simulink model "dqtransform2"  (R2014b)
settings: Solver=ode45  StartTime=0.0  StopTime=10  MaxStep=1e-4  RelTol=1e-3
undefined symbols (not defined in the file): f, Vg
settings Model: Creator=Iranga Weerasuriya  LastModifiedBy=ajunyent
settings DataIOCC: SignalLoggingSaveFormat=ModelDataLogs
settings DebuggingCC: MultiTaskDSMMsg=warning  MultiTaskCondExecSysMsg=none  StrictBusMsg=ErrorOnBusTreatedAsVector
settings RTWCC: IncludeERTFirstTime=on

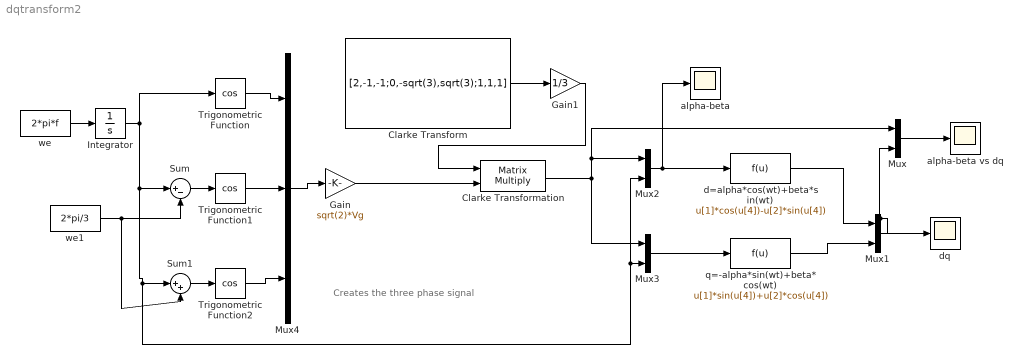
== system dqtransform2 ==
  note: Creates the three phase signal
  Clarke Transform : Constant  Value=[2,-1,-1;0,-sqrt(3),sqrt(3);1,1,1]
  Clarke Transformation : Product  Multiplication=Matrix(*)
  Gain : Gain  Gain=sqrt(2)*Vg
  Gain1 : Gain  Gain=1/3
  Integrator : Integrator
  Mux{,1..3} (4 alike) : Mux  Inputs=2
  Mux4 : Mux  Inputs=3
  Sum : Sum  Inputs=|+-
  Sum1 : Sum  Inputs=|++
  Trigonometric Function : Trigonometry  Operator=cos
  Trigonometric Function1 : Trigonometry  Operator=cos
  Trigonometric Function2 : Trigonometry  Operator=cos
  alpha-beta : Scope
      settings: ShowLegends=on  SaveName=ScopeData11
  alpha-beta vs dq : Scope
      settings: SaveName=ScopeData10
  d=alpha*cos(wt)+beta*sin(wt) : Fcn  Expr=u[1]*cos(u[4])-u[2]*sin(u[4])
  dq : Scope
  q=-alpha*sin(wt)+beta*cos(wt) : Fcn  Expr=u[1]*sin(u[4])+u[2]*cos(u[4])
  we : Constant  Value=2*pi*f
  we1 : Constant  Value=2*pi/3
  wires:
  we/1 -> Integrator/1
  Integrator/1 -> Mux3/2, Mux2/2, Sum1/1, Sum/1, Trigonometric Function/1
  Sum/1 -> Trigonometric Function1/1
  Sum1/1 -> Trigonometric Function2/1
  we1/1 -> Sum/2, Sum1/2
  Trigonometric Function/1 -> Mux4/1
  Trigonometric Function1/1 -> Mux4/2
  Trigonometric Function2/1 -> Mux4/3
  Mux4/1 -> Gain/1
  Clarke Transform/1 -> Gain1/1
  Gain1/1 -> Clarke Transformation/1
  Gain/1 -> Clarke Transformation/2
  Mux2/1 -> d=alpha*cos(wt)+beta*sin(wt)/1, alpha-beta/1
  Mux3/1 -> q=-alpha*sin(wt)+beta*cos(wt)/1
  d=alpha*cos(wt)+beta*sin(wt)/1 -> Mux1/1
  Mux1/1 -> Mux/2, dq/1
  q=-alpha*sin(wt)+beta*cos(wt)/1 -> Mux1/2
  Clarke Transformation/1 -> Mux3/1, Mux2/1, Mux/1
  Mux/1 -> alpha-beta vs dq/1
